simulink subsystem "XAxisSubsystem"  (R2023b)
settings: Solver=VariableStepAuto  StartTime=0.0  StopTime=10.0  RelTol=1e-3
values from neighbouring files (symbols this model uses):
  Ax = 0.0    (= 0)    [drone_input_params.m]
  m = weight/g    (= 0.815494393476)    [drone_input_params.m]
settings Model: Creator=FRESH  LastModifiedBy=FRESH

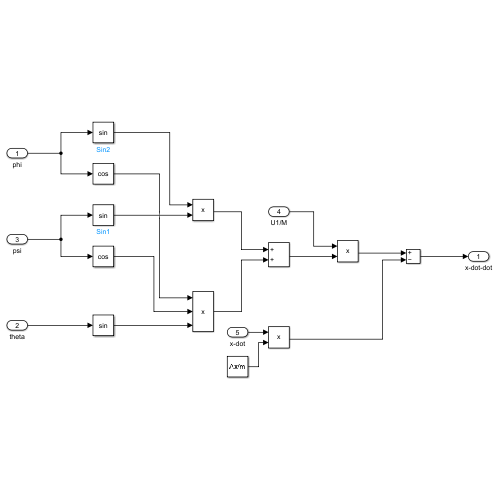
[thumbnail: Simulink's stored preview of the top-level diagram]
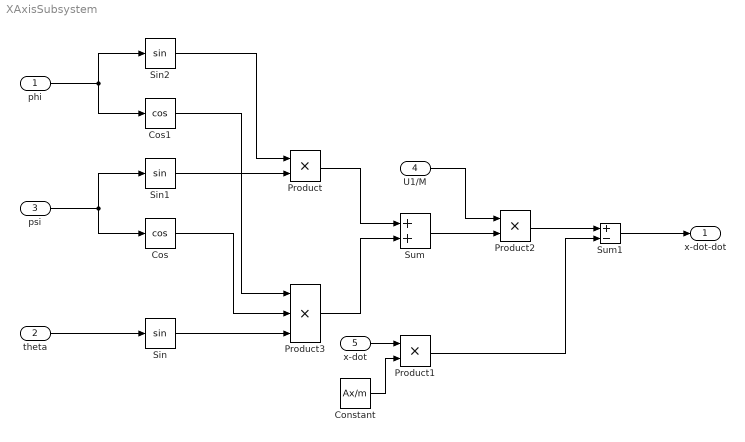
== system XAxisSubsystem ==
  phi : Inport
  theta : Inport  Port=2
  psi : Inport  Port=3
  U1/M : Inport  Port=4
  x-dot : Inport  Port=5
  Constant : Constant  Value=Ax/m
  Cos : Trigonometry  Operator=cos
  Cos1 : Trigonometry  Operator=cos
  Product : Product
  Product1 : Product
  Product2 : Product
  Product3 : Product  Inputs=3
  Sin : Trigonometry
  Sin1 : Trigonometry
  Sin2 : Trigonometry
  Sum : Sum
  Sum1 : Sum  Inputs=+-
  x-dot-dot : Outport
  wires:
  phi/1 -> Sin2/1, Cos1/1
  psi/1 -> Cos/1, Sin1/1
  theta/1 -> Sin/1
  Sin/1 -> Product3/3
  Cos/1 -> Product3/2
  Cos1/1 -> Product3/1
  Sin2/1 -> Product/1
  Sin1/1 -> Product/2
  Product/1 -> Sum/1
  Product3/1 -> Sum/2
  x-dot/1 -> Product1/1
  Constant/1 -> Product1/2
  Sum/1 -> Product2/2
  U1/M/1 -> Product2/1
  Product1/1 -> Sum1/2
  Product2/1 -> Sum1/1
  Sum1/1 -> x-dot-dot/1
